simulink model "Systeme"  (R2020a)
settings: Solver=VariableStepAuto  StartTime=0.0  StopTime=SimDuration  RelTol=1e-3  SampleTimeConstraint=Specified  EnableMultiTasking=on
values from neighbouring files (symbols this model uses):
  A = 10    [Config.m]
  BW = F_SC*N    (= 50000000)    [Config.m]
  F_US = BW/2    (= 25000000)    [Config.m]
  K = 960    [Config.m]
  M = N_FEC/t    (= 48)    [Config.m]
  N = 256    [Config.m]
  N_CP = N/4    (= 64)    [Config.m]
undefined symbols (not defined in the file or in its folder): BarkerCode, PreambleDetectorThreshold, qpsktxrx, R, SimDuration, SimSampleTime
libraries: commrflib2 x4, dspsigops x4, commsequence2 x3, commdigbbndam3 x3, commchan3 x2, simulink x2, dspxfrm3 x2, commutil2 x2, commblkcod2 x2, commrandsrc3 x1, commrfcorlib x1, dspstat3 x1
settings Model: Creator=Jsinno  LastModifiedBy=jsinno
settings DataIOCC: ReturnWorkspaceOutputs=off
settings OptimizationCC: LifeSpan=inf
settings DebuggingCC: SFUnexpectedBacktrackingDiag=warning  SFNoUnconditionalDefaultTransitionDiag=warning  ArithmeticOperatorsInVariantConditions=warning
settings SFSimCC: SimUseLocalCustomCode=off  CustomCodeUndefinedFunction=UseInterfaceOnly
settings RTWCC: RTWUseLocalCustomCode=off
settings CodeAppCC: StateflowObjectComments=on
settings GRTTargetCC: TargetLangStandard=C89/C90 (ANSI)
settings ConfigComp: CovMetricSettings=dw  CovHtmlReporting=on  CovSaveCumulativeToWorkspaceVar=on  CovSaveSingleToWorkspaceVar=on  CovExternalEMLEnable=off
settings SimscapeCC: SimscapeNormalizeSystem=off

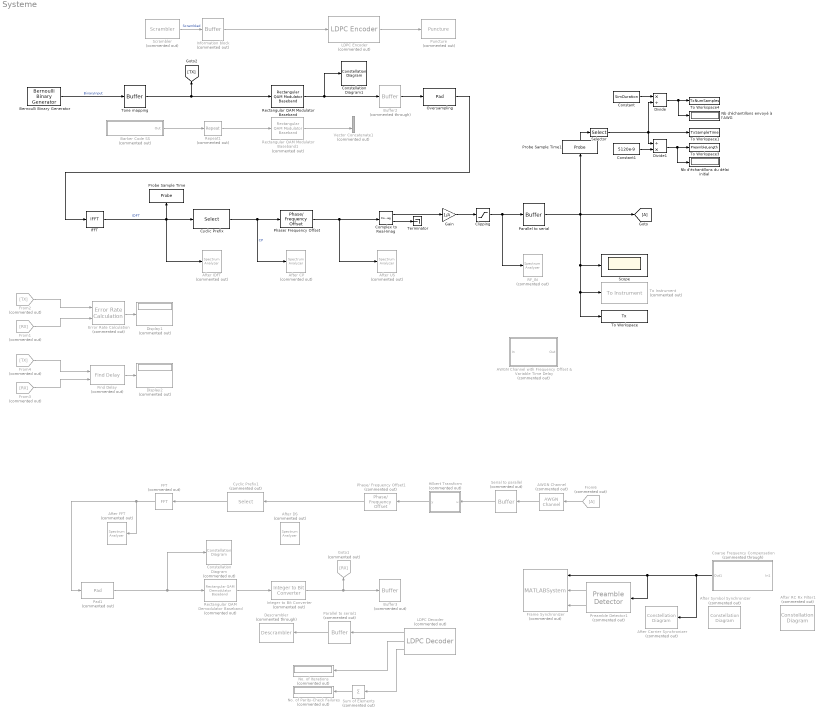
== system Systeme ==
  AWGN Channel : commchan3/AWGN Channel  Commented=on  InputProcessing=Columns as channels (frame based)  seed=2  noiseMode="Signal to noise ratio  (Eb/No)"  EbNodB=20  EsNodB=15  SNRdB=15  bitsPerSym=log2(qpsktxrx.ModulationOrder)  Ps=1/qpsktxrx.Interpolation  Tsym=qpsktxrx.Tsym  variance=1
  AWGN Channel with Frequency Offset & Variable Time Delay : Subsystem  Commented=on
      mask Display: disp('AWGN Channel with\nFrequency Offset & \nVariable Time Delay');
  After CP : SpectrumAnalyzer  Commented=on
  After Carrier Synchronizer : ConstellationDiagram  Tag=ScatterPlot  Commented=on
  After DS : SpectrumAnalyzer  Commented=on
  After FFT : SpectrumAnalyzer  Commented=on
  After IDFT : SpectrumAnalyzer  Commented=on
  After RC Rx Filter1 : ConstellationDiagram  Tag=ScatterPlot  Commented=on
  After Symbol Synchronizer : ConstellationDiagram  Tag=ScatterPlot  Commented=on
  After US : SpectrumAnalyzer  Commented=on
  Barker Code SS : Subsystem  Commented=on
      mask Display: disp('Unipolar\nBarker Code')
  Bernoulli Binary Generator : commrandsrc3/Bernoulli Binary Generator  ProbabilityOfZero=0.5  SeedSource=Auto  Seed=0  SampleTime=SimSampleTime  SamplesPerFrame=1  OutputDataType=boolean  SimulateUsing=Interpreted execution
  Buffer2 : Buffer  Commented=through  N=N  OutputFrames=off
  Buffer3 : Buffer  Commented=on  N=1920  OutputFrames=off
  Clipping : Saturate  UpperLimit=0.7  LowerLimit=-0.7
  Coarse Frequency Compensation : Subsystem  Commented=through
      mask Display: fprintf('Coarse Frequency\nCompensation')
  Complex to Real-Imag : ComplexToRealImag
  Constant : Constant  Value=SimDuration
  Constant1 : Constant  Value=5120e-9
  Constellation Diagram : ConstellationDiagram  Commented=on
  Constellation Diagram1 : ConstellationDiagram
  Cyclic Prefix : Selector  InputPortWidth=R*N  IndexOptions=Index vector (dialog)  Indices=[(R*N-R*N_CP+1):R*N 1:R*N]  OutputSizes=1
  Cyclic Prefix1 : Selector  Commented=on  InputPortWidth=R*N+N_CP  IndexOptions=Starting index (dialog)  Indices=N_CP+1  OutputSizes=R*N
  Descrambler : commsequence2/Descrambler  Commented=through  M=2  poly='1 + z^-18 + z^-23'  iniStaSource=Dialog Parameter  ini_sta=[1 1 1 1 1 1 1 1 1 1 1 1 1 1 1 1 1 1 1 1 1 1 1]  resetViaPort=off
      settings: SourceProductBaseCode=CM
  Display1 : Display  Commented=on
  Display2 : Display  Commented=on
      settings: Decimation=2
  Divide : Product  Inputs=*/
  Divide1 : Product  Inputs=/*
  Error Rate Calculation : commsink2/Error Rate Calculation  Commented=on  N=2*N  st_delay=0  cp_mode=Entire frame  subframe=[]  PMode=Port  WsName=ErrorVec  RsMode2=off  stop=on  numErr=100  maxBits=1e6
  FFT : dspxfrm3/FFT  Commented=on  FFTImplementation=Auto  CompMethod=Table lookup  TableOpt=NEW  TableOptActive=Speed  BitRevOrder=off  Normalize=off  InheritFFTLength=on  FFTLength=64  WrapInput=on  roundingMode=Floor  overflowMode=off  firstCoeffDataTypeStr=Inherit: Same word length as input  firstCoeffLastDataTypeStr=Inherit: Same word length as input  outputMin=[]  outputMax=[]
  Find Delay : commutil2/Find Delay  Commented=on  corrLength=2*N+4*K  chgSigOP=off  stopUpdate=off  numConstDelay=3
      settings: SourceProductBaseCode=CM
  Frame Synchronizer : MATLABSystem  Commented=on  System=comm.internal.examples.FrameSynchronizer  Input=Symbol  OutputFrameLength=R*N+N_CP  PreambleLength=BarkerLength  SimulateUsing=Code generation
      mask Type: comm.internal.examples.FrameSynchronizer
      mask Display:
      | disp(['Frame' char(10) 'Synchronizer']);
      | port_label('input',1,'u');
      | port_label('input',2,'idx');
      | port_label('input',3,'dtMt');
      | port_label('output',1,'Frame');
      | port_label('output',2,'Valid');
  From1 : From  Commented=on  GotoTag=RX
  From2 : From  Commented=on  GotoTag=TX
  From3 : From  Commented=on  GotoTag=RX
  From4 : From  Commented=on  GotoTag=TX
  From6 : From  Commented=on
  Gain : Gain  Gain=1/A
  Goto1 : Goto  Commented=on  GotoTag=RX
  Hilbert Transform : MATLAB Function  Commented=on  TreatAsAtomicUnit=on
  IFFT : dspxfrm3/IFFT  FFTImplementation=Auto  CompMethod=Table lookup  TableOpt=NEW  TableOptActive=Speed  BitRevOrder=off  cs_in=off  Normalize=off  InheritFFTLength=on  FFTLength=R*N  WrapInput=off  mode=Complex  outSamplingMode=Sample based  roundingMode=Floor  overflowMode=off  firstCoeffDataTypeStr=Inherit: Same word length as input  firstCoeffLastDataTypeStr=Inherit: Same word length as input  outputMin=[]  outputMax=[]
  Information block : Buffer  Commented=on  N=K  OutputFrames=off
  Integer to Bit Converter : commutil2/Integer to Bit Converter  Commented=on  nbits=log2(M)  signedInputValues=Unsigned  bitOrder=MSB first  outDtype=boolean
  LDPC Decoder : commblkcod2/LDPC Decoder  Commented=on  ParityCheckMat=H  OutputFmt=Information part  DecisionType=Hard decision  OutputDataType=boolean  NumIter=100  DoParityCheck=on  OutputNumIter=on  OutputFinalChecks=on
      settings: SourceProductBaseCode=CM
  LDPC Encoder : commblkcod2/LDPC Encoder  Commented=on  ParityCheckMat=H
      settings: SourceProductBaseCode=CM
  Nb d'échantillons du délai initial : Display
  Nb d'échantillons envoyé à l'AWG : Display
  No. of Iterations : Display  Commented=on
  No. of Parity-Check Failures : Display  Commented=on
  Oversampling : dspsigops/Pad  padAlong=Columns  dimsToPad=1  valSrc=Specify via dialog  padVal=0  spec=Output size  padNumOutRowsSpecMethod=User-specified  numOutRows=R*N  padNumOutColsSpecMethod=User-specified  numOutCols=256  isVarDimsMode=off  padBeginning=0  padEnd=0  outSizeMode=User-specified  outSize=1  padSigAt=Beginning and end  trunc_flag=None  roundingMode=Floor  overflowMode=off  truncOrWrapMode=Truncate  wrap_flag=None
      settings: SourceProductBaseCode=DS
  Pad1 : dspsigops/Pad  Commented=on  padAlong=Columns  dimsToPad=1  valSrc=Specify via dialog  padVal=0  spec=Output size  padNumOutRowsSpecMethod=User-specified  numOutRows=N  padNumOutColsSpecMethod=User-specified  numOutCols=256  isVarDimsMode=off  padBeginning=0  padEnd=0  outSizeMode=User-specified  outSize=1  padSigAt=Beginning and end  trunc_flag=None  roundingMode=Floor  overflowMode=off  truncOrWrapMode=Truncate  wrap_flag=None
      settings: SourceProductBaseCode=DS
  Parallel to serial : Buffer  N=1  OutputFrames=off
  Parallel to serial1 : Buffer  Commented=on  N=1  OutputFrames=off
  Phase/ Frequency Offset : commrflib2/Phase// Frequency Offset  phaseOffset=0  freqPort=off  freqOffset=R*BW/2+F_US
  Phase/ Frequency Offset1 : commrflib2/Phase// Frequency Offset  Commented=on  phaseOffset=0  freqPort=off  freqOffset=-(R*BW/2+F_US)
  Preamble Detector1 : commsync2/Preamble Detector  Commented=on  Input=Symbol  Preamble=sqrt(2)/2 * (-1-1i) * (BarkerCode)'  Threshold=PreambleDetectorThreshold  DetectionMetricOutput=on  Detections=All  SimulateUsing=Code generation
      settings: SourceProductBaseCode=CM
  Probe Sample Time : Probe  ProbeWidth=off  ProbeComplexSignal=off
  Probe Sample Time1 : Probe  ProbeWidth=off  ProbeComplexSignal=off
  Puncture : commsequence2/Puncture  Commented=on  punctureVector=[1 1 1 1 1 1 1 1 1 1 1 1 1 1 1 1] .'
      settings: SourceProductBaseCode=CM
  RF_IN : SpectrumAnalyzer  Commented=on
  Rectangular QAM Demodulator Baseband : commdigbbndam3/Rectangular QAM Demodulator Baseband  Commented=on  M=M  OutType=Integer  DecType=Hard decision  VarSource=Dialog  Variance=1  Dec=Gray  Mapping=[0:15]  PowType=Average Power  MinDist=2  AvgPow=50  PeakPow=1  Ph=-pi/11  outDtype1=Inherit via internal rule  outDtype2=double  derotateFactorWordLen=16  derotateFactorDataTypeStr=Inherit: Same word length as input  derotateFactorLastDataTypeStr=Inherit: Same word length as input  denormFactorWordLen=16  denormFactorDataTypeStr=Inherit: Same word length as input  denormFactorLastDataTypeStr=Inherit: Same word length as input  prodOutWordLen=32  prodOutOverflowMode=Wrap  prodOutRoundingMode=Floor  prodOutOvFlMode=off  prodOutOvFlModeLastStrValue=off  sumWordLen=32
  Rectangular QAM Modulator Baseband : commdigbbndam3/Rectangular QAM Modulator Baseband  M=M  InType=Bit  Enc=Gray  Mapping=[0:15]  PowType=Average Power  MinDist=2  AvgPow=1  PeakPow=1  Ph=0  outDtype=double  outWordLen=16  outUDDataType=sfix(16)  outFracLenMode=Best precision  outFracLen=15  outDataTypeStr=double  outLastDataTypeStr=double
  Rectangular QAM Modulator Baseband1 : commdigbbndam3/Rectangular QAM Modulator Baseband  Commented=on  M=16  InType=Bit  Enc=Gray  Mapping=[0:15]  PowType=Average Power  MinDist=2  AvgPow=1  PeakPow=1  Ph=0  outDtype=double  outWordLen=16  outUDDataType=sfix(16)  outFracLenMode=Best precision  outFracLen=15  outDataTypeStr=double  outLastDataTypeStr=double
  Repeat1 : dspsigops/Repeat  Commented=on  N=8  InputProcessing=Columns as channels (frame based)  RateOptions=Enforce single-rate processing  ic=0  mode=Unused parameter value
  Scope : Scope
  Scrambler : commsequence2/Scrambler  Commented=on  M=2  poly='1 + z^-18 + z^-23'  iniStaSource=Dialog Parameter  ini_sta=[1 1 1 1 1 1 1 1 1 1 1 1 1 1 1 1 1 1 1 1 1 1 1]  resetViaPort=off
      settings: SourceProductBaseCode=CM
  Selector : Selector  InputPortWidth=2  IndexOptions=Index vector (dialog)  Indices=[1]  OutputSizes=1
  Serial to parallel : Buffer  Commented=on  N=R*N+N_CP  OutputFrames=off
  Sum of Elements : Sum  Commented=on  Inputs=+
  Terminator : Terminator
  To Instrument : instrumentlib/To Instrument  Commented=on  sampleTime=-1  isWorkspaceObject=off  timeout=10  inputBufferSize=8192  protocol=VISA USB  serialPort=COM1  baudRate=9600  gpibVendor=ICS Electronics  boardIndex=0  primaryAddress=1  secondaryAddress=0  visaVendor=Keysight  visaSerialPort=0  chassisIndex=0  logicalAddress=0  tcpRemoteHost='127.0.0.1'  tcpRemotePort=4500  udpRemoteHost='127.0.0.1'  udpRemotePort=9090  visaTCPBoardIndex=0  visaTCPRemoteHost='127.0.0.1'  usbBoardIndex=0  usbManufID=0  usbModelCode=0  usbSerialNumber=0  initAction=None  initCommand='DATA:SOURCE CH1'  initFunction=get  command=''  sendFormat=ASCII  asciiFormatting='%d'  precision=8-bit integer  byteOrder=Little endian
      settings: SourceProductBaseCode=IC
  To Workspace : ToWorkspace  VariableName=Tx  SaveFormat=Timeseries  SampleTime=-1
      settings: Save2DSignal=2-D array (concatenate along first dimension)
  To Workspace1 : ToWorkspace  VariableName=TxSampleTime  SampleTime=-1
      settings: MaxDataPoints=1  Save2DSignal=2-D array (concatenate along first dimension)
  To Workspace3 : ToWorkspace  VariableName=PreambleLength  SampleTime=-1
      settings: MaxDataPoints=1  Save2DSignal=2-D array (concatenate along first dimension)
  To Workspace4 : ToWorkspace  VariableName=TxNumSamples  SampleTime=-1
      settings: MaxDataPoints=1  Save2DSignal=2-D array (concatenate along first dimension)
  Tone mapping : Buffer  N=N*log2(M)  OutputFrames=off
  Vector Concatenate1 : Concatenate  Commented=on
  wires:
  Rectangular QAM Modulator Baseband/1 -> Constellation Diagram1/1, Buffer2/1
  LDPC Encoder/1 -> Puncture/1
  Scrambler/1 -> Information block/1  "Scrambled"
  IFFT/1 -> Probe Sample Time/1, Cyclic Prefix/1, After IDFT/1  "IDFT"
  Cyclic Prefix1/1 -> FFT/1
  Complex to Real-Imag/2 -> Terminator/1
  Find Delay/1 -> Display2/1
  Error Rate Calculation/1 -> Display1/1
  Phase/ Frequency Offset/1 -> Complex to Real-Imag/1, After US/1
  FFT/1 -> After FFT/1, Pad1/1
  Hilbert Transform/1(y) -> Phase/ Frequency Offset1/1
  Cyclic Prefix/1 -> Phase/ Frequency Offset/1, After CP/1  "CP"
  Complex to Real-Imag/1 -> Gain/1
  From1/1 -> Error Rate Calculation/2
  From2/1 -> Error Rate Calculation/1
  From4/1 -> Find Delay/1
  From3/1 -> Find Delay/2
  LDPC Decoder/1 -> Parallel to serial1/1
  Parallel to serial1/1 -> Descrambler/1
  Sum of Elements/1 -> No. of Parity-Check Failures/1
  LDPC Decoder/2 -> No. of Iterations/1
  LDPC Decoder/3 -> Sum of Elements/1
  Coarse Frequency Compensation/1(Out1) -> Frame Synchronizer/1, Preamble Detector1/1, After Carrier Synchronizer/1
  Preamble Detector1/1 -> Frame Synchronizer/2
  Preamble Detector1/2 -> Frame Synchronizer/3
  Information block/1 -> LDPC Encoder/1
  Oversampling/1 -> IFFT/1
  Serial to parallel/1 -> Hilbert Transform/1(u)
  Rectangular QAM Demodulator Baseband/1 -> Integer to Bit Converter/1
  Integer to Bit Converter/1 -> Goto1/1, Buffer3/1
  Barker Code SS/1(Out) -> Repeat1/1
  Repeat1/1 -> Rectangular QAM Modulator Baseband1/1
  Buffer2/1 -> Oversampling/1
  Phase/ Frequency Offset1/1 -> Cyclic Prefix1/1
  Rectangular QAM Modulator Baseband1/1 -> Vector Concatenate1/2
  Tone mapping/1 -> Rectangular QAM Modulator Baseband/1, [TX]
  Pad1/1 -> Rectangular QAM Demodulator Baseband/1, Constellation Diagram/1
  From6/1 -> AWGN Channel/1
  AWGN Channel/1 -> Serial to parallel/1
  Bernoulli Binary Generator/1 -> Tone mapping/1  "BinaryInput"
  Gain/1 -> Clipping/1
  Parallel to serial/1 -> Scope/1, To Workspace/1, To Instrument/1, [A], Probe Sample Time1/1
  Clipping/1 -> RF_IN/1, Parallel to serial/1
  Probe Sample Time1/1 -> Selector/1
  Constant/1 -> Divide/1
  Divide/1 -> To Workspace4/1, Nb d'échantillons envoyé à l'AWG/1
  Selector/1 -> Divide1/1, Divide/2, To Workspace1/1
  Constant1/1 -> Divide1/2
  Divide1/1 -> To Workspace3/1, Nb d'échantillons du délai initial/1

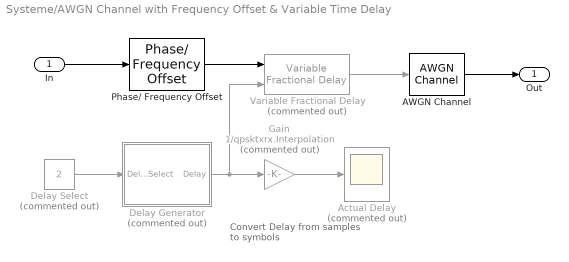
== system Systeme/AWGN Channel with Frequency Offset & Variable Time Delay ==
  note: Convert Delay from
      | samples to symbols
  In : Inport
  AWGN Channel : commchan3/AWGN Channel  InputProcessing=Columns as channels (frame based)  seed=2  noiseMode="Signal to noise ratio  (Eb/No)"  EbNodB=20  EsNodB=15  SNRdB=15  bitsPerSym=log2(qpsktxrx.ModulationOrder)  Ps=1/qpsktxrx.Interpolation  Tsym=qpsktxrx.Tsym  variance=1
  Actual Delay : Scope  Commented=on
  Delay Generator : Subsystem  Commented=on
      mask Display: disp('Delay Generator')
  Delay Select : Constant  Commented=on  Value=2
  Gain : Gain  Commented=on  Gain=1/qpsktxrx.Interpolation
  Phase/ Frequency Offset : commrflib2/Phase// Frequency Offset  phaseOffset=47  freqPort=off  freqOffset=5000
  Variable Fractional Delay : dspsigops/Variable Fractional Delay  Commented=on  mode=OBSOLETE  modeActive=Linear  L=4  FarrowL=4  R=10  alpha=1  dmax=qpsktxrx.FrameSize*qpsktxrx.Interpolation  InputProcessing=Columns as channels (frame based)  ic=0  noDFT=off  fallbackFIR=Clip to the minimum value necessary for centered kernel  fallbackFarrow=Clip to the minimum value necessary for centered kernel  roundingMode=Zero  overflowMode=off
      settings: SourceProductBaseCode=DS
  Out : Outport  VectorParamsAs1DForOutWhenUnconnected=off
  wires:
  AWGN Channel/1 -> Out/1
  In/1 -> Phase/ Frequency Offset/1
  Delay Select/1 -> Delay Generator/1(Delay Select)
  Delay Generator/1(Delay) -> Variable Fractional Delay/2, Gain/1
  Gain/1 -> Actual Delay/1
  Phase/ Frequency Offset/1 -> Variable Fractional Delay/1
  Variable Fractional Delay/1 -> AWGN Channel/1

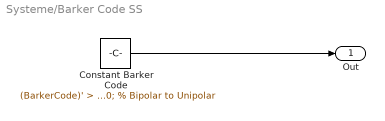
== system Systeme/Barker Code SS ==
  Constant Barker Code : Constant  Value=(BarkerCode)' > 0; % Bipolar to Unipolar  VectorParams1D=off  OutDataTypeStr=boolean  SampleTime=Inf
  Out : Outport  VectorParamsAs1DForOutWhenUnconnected=off
  wires:
  Constant Barker Code/1 -> Out/1

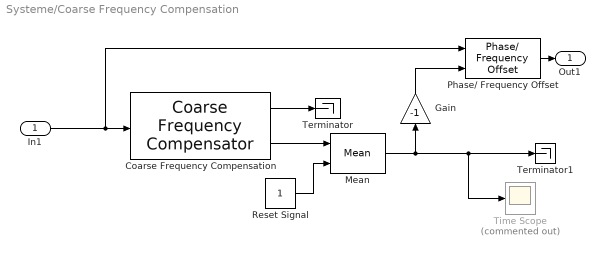
== system Systeme/Coarse Frequency Compensation ==
  In1 : Inport
  Coarse Frequency Compensation : commrfcorlib/Coarse Frequency Compensator  Modulation=QPSK  Algorithm=Correlation-based  FrequencyResolution=25  MaximumFrequencyOffset=1000  SamplesPerSymbol=4  EstimatedFreqOffsetPort=on  SimulateUsing=Code generation
      settings: SourceProductBaseCode=CM
  Gain : Gain  Gain=-1
  Mean : dspstat3/Mean  run=on  InputProcessing=Columns as channels (frame based)  reset_popup=Either edge  directionMode=Each column  dimension=1  roiEnable=off  roiType=Rectangles  roiPortion=Entire ROI  roiOutput=Individual statistics for each ROI  roiFlag=off  roundingMode=Floor  overflowMode=off  outputDataTypeStr=Inherit: Same as accumulator  outputMin=[]  outputMax=[]  outputLastDataTypeStr=Inherit: Same as accumulator
  Phase/ Frequency Offset : commrflib2/Phase// Frequency Offset  phaseOffset=0  freqPort=on  freqOffset=0
  Reset Signal : Constant
  Terminator : Terminator
  Terminator1 : Terminator
  Time Scope : Scope  Commented=on
  Out1 : Outport  VectorParamsAs1DForOutWhenUnconnected=off
  wires:
  In1/1 -> Phase/ Frequency Offset/1, Coarse Frequency Compensation/1
  Phase/ Frequency Offset/1 -> Out1/1
  Mean/1 -> Time Scope/1, Terminator1/1, Gain/1
  Coarse Frequency Compensation/2 -> Mean/1
  Coarse Frequency Compensation/1 -> Terminator/1
  Gain/1 -> Phase/ Frequency Offset/2
  Reset Signal/1 -> Mean/2

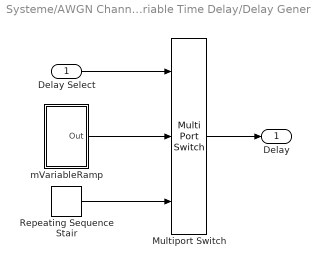
== system Systeme/AWGN Channel with Frequency Offset & Variable Time Delay/Delay Generator ==
  Delay Select : Inport
  Multiport Switch : MultiPortSwitch  Inputs=2  OutDataTypeStr=double
  Repeating Sequence Stair : simulink/Sources/Repeating Sequence Stair  OutValues="[0       0.025        0.05       0.075         0.1       0.125        0.15       0.175         0.2       0.225        0.25       0.275         0.3       0.325        0.35       0.375         0.4       0.425        0.45       0.475         0.5       0.525        0.55       0.575         0.6       0.625        0.65       0.675         0.7       0.725        0.75       0.775         0.8       0.825        0.85       0.875         0.9       0.925        0.95       0.975           1       1.025        1.05       1.075         1.1       1.125        1.15       1.175         1.2       1.225        1.25       1.275         1.3       1.325        1.35       1.375         1.4       1.425        1.45       1.475         1.5       1.525        1.55       1.575         1.6       1.625        1.65       1.675         1.7       1.725        1.75       1.775         1.8       1.825        1.85       1.875         1.9       1.925        1.95       1.975           2       2.025        2.05       2.075         2.1       2.125        2.15       2.175         2.2       2.225        2.25       2.275         2.3       2.325        2.35       2.375         2.4       2.425        2.45       2.475         2.5       2.525        2.55       2.575         2.6       2.625        2.65       2.675         2.7       2.725        2.75       2.775         2.8       2.825        2.85       2.875         2.9       2.925        2.95       2.975           3       3.025        3.05       3.075         3.1       3.125        3.15       3.175         3.2       3.225        3.25       3.275         3.3       3.325        3.35       3.375         3.4       3.425        3.45       3.475         3.5       3.525        3.55       3.575         3.6       3.625        3.65       3.675         3.7       3.725        3.75       3.775         3.8       3.825        3.85       3.875         3.9       3.925        3.95       3.975           4       3.975        3.95       3.925         3.9       3.875        3.85       3.825         3.8       3.775        3.75       3.725         3.7       3.675        3.65       3.625         3.6       3.575        3.55       3.525         3.5       3.475        3.45       3.425         3.4       3.375        3.35       3.325         3.3       3.275        3.25       3.225         3.2       3.175        3.15       3.125         3.1       3.075        3.05       3.025           3       2.975        2.95       2.925         2.9       2.875        2.85       2.825         2.8       2.775        2.75       2.725         2.7       2.675        2.65       2.625         2.6       2.575        2.55       2.525         2.5       2.475        2.45       2.425         2.4       2.375        2.35       2.325         2.3       2.275        2.25       2.225         2.2       2.175        2.15       2.125         2.1       2.075        2.05       2.025           2       1.975        1.95       1.925         1.9       1.875        1.85       1.825         1.8       1.775        1.75       1.725         1.7       1.675        1.65       1.625         1.6       1.575        1.55       1.525         1.5       1.475        1.45       1.425         1.4       1.375        1.35       1.325         1.3       1.275        1.25       1.225         1.2       1.175        1.15       1.125         1.1       1.075        1.05       1.025           1       0.975        0.95       0.925         0.9       0.875        0.85       0.825         0.8       0.775        0.75       0.725         0.7       0.675        0.65       0.625         0.6       0.575        0.55       0.525         0.5       0.475        0.45       0.425         0.4       0.375        0.35       0.325         0.3       0.275        0.25       0.225         0.2       0.175        0.15       0.125         0.1       0.075        0.05       0.025]"  tsamp=qpsktxrx.FrameTime  OutMin=[]  OutMax=[]  OutDataTypeStr=double  OutputDataTypeScalingMode=double  OutDataType=fixdt(0,8)  ConRadixGroup=Best Precision: Vector-wise  OutScaling=2^-12
  mVariableRamp : Subsystem
  Delay : Outport  VectorParamsAs1DForOutWhenUnconnected=off
  wires:
  Delay Select/1 -> Multiport Switch/1
  Repeating Sequence Stair/1 -> Multiport Switch/3
  mVariableRamp/1(Out) -> Multiport Switch/2
  Multiport Switch/1 -> Delay/1

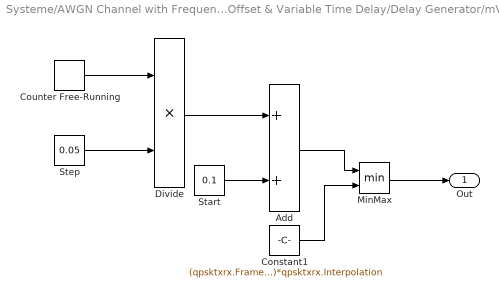
== system Systeme/AWGN Channel with Frequency Offset & Variable Time Delay/Delay Generator/mVariableRamp ==
  Add : Sum
  Constant1 : Constant  Value=(qpsktxrx.FrameSize-qpsktxrx.RaisedCosineFilterSpan)*qpsktxrx.Interpolation
  Counter Free-Running : simulink/Sources/Counter Free-Running  NumBits=64  tsamp=qpsktxrx.FrameTime
  Divide : Product  Inputs=**
  MinMax : MinMax  Inputs=2
  Start : Constant  Value=0.1
  Step : Constant  Value=0.05
  Out : Outport  VectorParamsAs1DForOutWhenUnconnected=off
  wires:
  Counter Free-Running/1 -> Divide/1
  Step/1 -> Divide/2
  Divide/1 -> Add/1
  Start/1 -> Add/2
  Add/1 -> MinMax/1
  MinMax/1 -> Out/1
  Constant1/1 -> MinMax/2

== matlab function Systeme/Hilbert Transform ==
  data: u input; y output
function y = fcn(u)

y = hilbert(u);
